simulink subsystem "TwoActuatorAWD"  (R2025b)
settings: Solver=VariableStepAuto  StartTime=0.0  StopTime=10.0  RelTol=1e-3
settings Model: Creator=The MathWorks, Inc.  LastModifiedBy=The MathWorks, Inc.
settings RTWCC: GPUComputeCapability=3.5

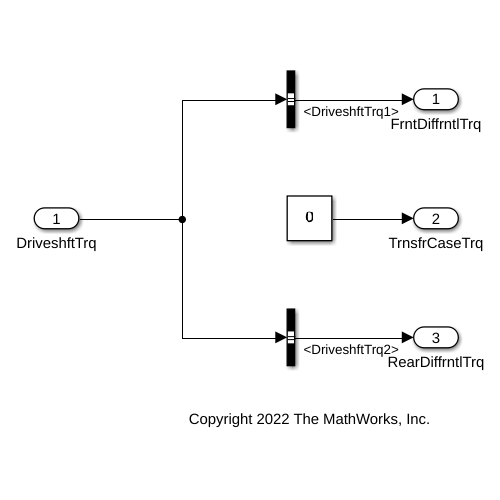
[thumbnail: Simulink's stored preview of the top-level diagram]
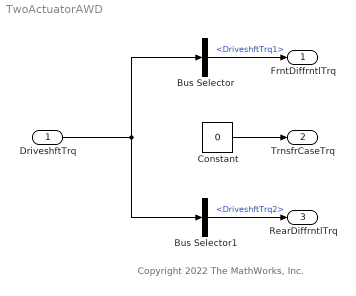
== system TwoActuatorAWD ==
  note: Copyright 2022 The MathWorks, Inc.
  DriveshftTrq : Inport
  Bus Selector : BusSelector  OutputSignals=DriveshftTrq1
  Bus Selector1 : BusSelector  OutputSignals=DriveshftTrq2
  Constant : Constant  Value=0  SampleTime=-1
  FrntDiffrntlTrq : Outport
  TrnsfrCaseTrq : Outport  Port=2
  RearDiffrntlTrq : Outport  Port=3
  wires:
  Bus Selector1/1 -> RearDiffrntlTrq/1  "<DriveshftTrq2>"
  DriveshftTrq/1 -> Bus Selector/1, Bus Selector1/1
  Bus Selector/1 -> FrntDiffrntlTrq/1  "<DriveshftTrq1>"
  Constant/1 -> TrnsfrCaseTrq/1
